simulink model "bench_native_plant"  (R2024b)
settings: Solver=daessc  StartTime=0.0  StopTime=60  MaxStep=1e-2  RelTol=1e-3
libraries: loco_native_lib x1
settings Model: Creator=BillBeverley  LastModifiedBy=BillBeverley

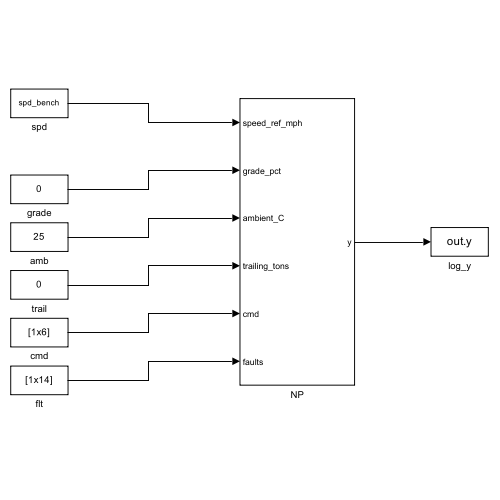
[thumbnail: Simulink's stored preview of the top-level diagram]
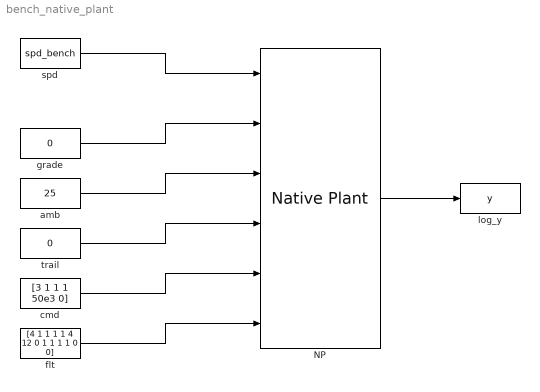
== system bench_native_plant ==
  NP : loco_native_lib/Native Plant  SystemSampleTime=-1  VariantActivationTime=update diagram  AllowFlexibleInterface=on  Latency=0  AutoFrameSizeCalculation=off
  amb : Constant  Value=25
  cmd : Constant  Value=[3 1 1 1 50e3 0]
  flt : Constant  Value=[4 1 1 1 1 4 12 0 1 1 1 1 0 0]
  grade : Constant  Value=0
  log_y : ToWorkspace  VariableName=y  SaveFormat=Timeseries  SampleTime=-1
  spd : FromWorkspace  VariableName=spd_bench
  trail : Constant  Value=0
  wires:
  grade/1 -> NP/2
  amb/1 -> NP/3
  trail/1 -> NP/4
  cmd/1 -> NP/5
  flt/1 -> NP/6
  spd/1 -> NP/1
  NP/1 -> log_y/1
